simulink model "PID_DC_MOTOR"  (R2016a)
settings: Solver=VariableStepAuto  StartTime=0.0  StopTime=tfinal  RelTol=1e-3
InitFcn:
  | J = 0.02;
  | b = 0.05;
  | Ke = 0.1;
  | Kt = 0.2;
  | R = 3;
  | L = 0.5;
  | 
  | thetha_dot0 = 0;
  | i0 = 0;
  | 
values from neighbouring files (symbols this model uses):
  Kd = 0.154298043345485    (= 0.154298043345)    [PID_DC_motor.m]
  Ki = 3.79137917089873    (= 3.7913791709)    [PID_DC_motor.m]
  Kp = 1.58461932315823    (= 1.58461932316)    [PID_DC_motor.m]
libraries: simulink x1
settings Model: Creator=hp  LastModifiedBy=hp

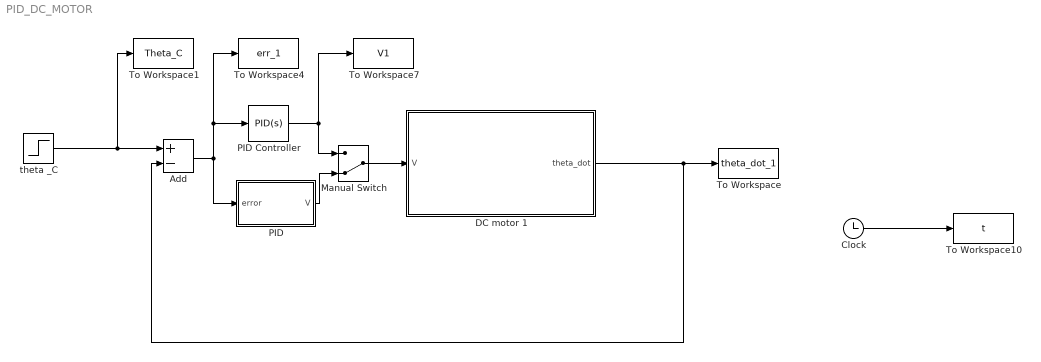
== system PID_DC_MOTOR ==
  Add : Sum  Inputs=+-
  Clock : Clock
  DC motor 1 : Subsystem
  Manual Switch : ManualSwitch  CurrentSetting=0
  PID : Subsystem
  "PID Controller " : simulink/Continuous/PID Controller  Controller=PID  TimeDomain=Continuous-time  SampleTime=-1  IntegratorMethod=Forward Euler  FilterMethod=Forward Euler  Form=Parallel  UseFilter=on  ControllerParametersSource=internal  P=1.58461932315823  I=3.79137917089873  D=0.154298043345485  N=439.358617384515  InitialConditionSource=internal  InitialConditionForIntegrator=0  InitialConditionForFilter=0  ExternalReset=none  LimitOutput=off  UpperSaturationLimit=inf  LowerSaturationLimit=-inf  LinearizeAsGain=on  AntiWindupMode=none  Kb=1  TrackingMode=off  Kt=1  PParamMin=[]  PParamMax=[]  IParamMin=[]  IParamMax=[]  DParamMin=[]  DParamMax=[]  NParamMin=[]  NParamMax=[]  KbParamMin=[]  KbParamMax=[]  KtParamMin=[]  KtParamMax=[]  POutMin=[]  POutMax=[]  IOutMin=[]  IOutMax=[]  DOutMin=[]  DOutMax=[]  NOutMin=[]  NOutMax=[]  KbOutMin=[]  KbOutMax=[]  KtOutMin=[]  KtOutMax=[]  IntegratorOutMin=[]  IntegratorOutMax=[]  FilterOutMin=[]  FilterOutMax=[]  SumOutMin=[]  SumOutMax=[]  SumI1OutMin=[]  SumI1OutMax=[]  SumI2OutMin=[]  SumI2OutMax=[]  SumI3OutMin=[]  SumI3OutMax=[]  SumDOutMin=[]  SumDOutMax=[]  SaturationOutMin=[]  SaturationOutMax=[]  IntegratorContinuousStateAttributes=''  IntegratorStateMustResolveToSignalObject=off  IntegratorRTWStateStorageClass=Auto  FilterContinuousStateAttributes=''  FilterStateMustResolveToSignalObject=off  FilterRTWStateStorageClass=Auto  DifferentiatorICPrevScaledInput=0  DifferentiatorOutMin=[]  DifferentiatorOutMax=[]
  To Workspace : ToWorkspace  VariableName=theta_dot_1  SampleTime=-1
  To Workspace1 : ToWorkspace  VariableName=Theta_C  SampleTime=-1
  To Workspace10 : ToWorkspace  VariableName=t  SampleTime=-1
      settings: Save2DSignal=2-D array (concatenate along first dimension)
  To Workspace4 : ToWorkspace  VariableName=err_1  SampleTime=-1
  To Workspace7 : ToWorkspace  VariableName=V1  SampleTime=-1
  theta _C : Step  Time=0  After=0.25  SampleTime=0
  wires:
  DC motor 1/1(theta_dot) -> Add/2, To Workspace/1
  "PID Controller "/1 -> Manual Switch/1, To Workspace7/1
  Add/1 -> PID/1(error), To Workspace4/1, "PID Controller "/1
  theta _C/1 -> Add/1, To Workspace1/1
  Clock/1 -> To Workspace10/1
  PID/1(V) -> Manual Switch/2
  Manual Switch/1 -> DC motor 1/1(V)

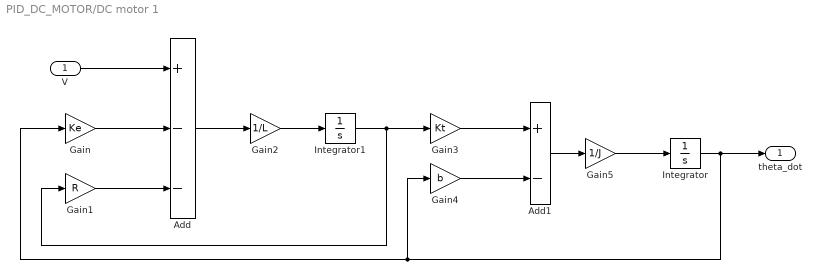
== system PID_DC_MOTOR/DC motor 1 ==
  V : Inport
  Add : Sum  Inputs=+--
  Add1 : Sum  Inputs=+-
  Gain : Gain  Gain=Ke
  Gain1 : Gain  Gain=R
  Gain2 : Gain  Gain=1/L
  Gain3 : Gain  Gain=Kt
  Gain4 : Gain  Gain=b
  Gain5 : Gain  Gain=1/J
  Integrator : Integrator  InitialCondition=thetha_dot0
  Integrator1 : Integrator  InitialCondition=i0
  theta_dot : Outport
  wires:
  Integrator/1 -> theta_dot/1, Gain4/1, Gain/1
  V/1 -> Add/1
  Gain5/1 -> Integrator/1
  Gain3/1 -> Add1/1
  Gain2/1 -> Integrator1/1
  Gain1/1 -> Add/3
  Add/1 -> Gain2/1
  Add1/1 -> Gain5/1
  Gain4/1 -> Add1/2
  Integrator1/1 -> Gain1/1, Gain3/1
  Gain/1 -> Add/2

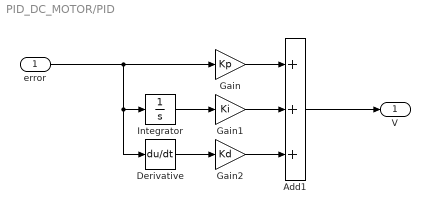
== system PID_DC_MOTOR/PID ==
  error : Inport
  Add1 : Sum  Inputs=+++
  Derivative : Derivative
  Gain : Gain  Gain=Kp
  Gain1 : Gain  Gain=Ki
  Gain2 : Gain  Gain=Kd
  Integrator : Integrator
  V : Outport
  wires:
  error/1 -> Derivative/1, Integrator/1, Gain/1
  Add1/1 -> V/1
  Gain/1 -> Add1/1
  Gain1/1 -> Add1/2
  Derivative/1 -> Gain2/1
  Gain2/1 -> Add1/3
  Integrator/1 -> Gain1/1
